simulink model "Powertrain_model"  (R2021b)
settings: Solver=VariableStepAuto  StartTime=0.0  StopTime=1220  RelTol=1e-3
values from neighbouring files (symbols this model uses):
  DR = 5.213    [Sim_script.m]    (also in workspace.mat)
  MaxLimit = [2.1951    294.39 ... (first row only)    [power_distribute_func.m]
  P_CE_idle = 0    [Sim_script.m]    (also in workspace.mat = 1)
  Trans_In = 24.086    [Sim_script.m]    (also in workspace.mat)
  w_CE_idle = 400    [Sim_script.m]    (also in workspace.mat = 32)
undefined symbols (not defined in the file or in its folder): dt, ENABLE_FUEL_CUTOFF, Fuel_con_map, H_u, P_CE_cutoff, Res_Torque, RPM_Load, T_CE_cutoff, T_CE_max, theta_CE, time, w_CE_max, w_CE_upper
libraries: visionstatistics x1, slpidlib x1
settings Model: Creator=Sagar Singhal  LastModifiedBy=Sagar Singhal

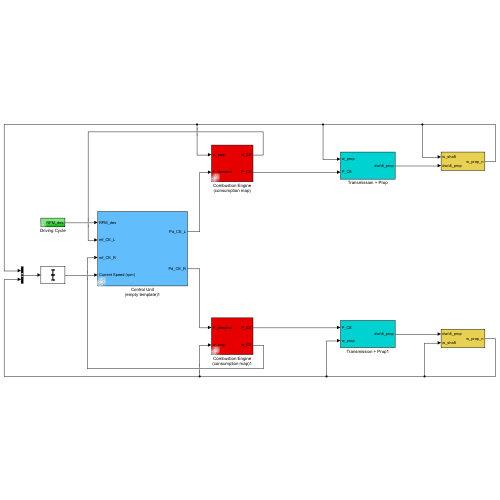
[thumbnail: Simulink's stored preview of the top-level diagram]
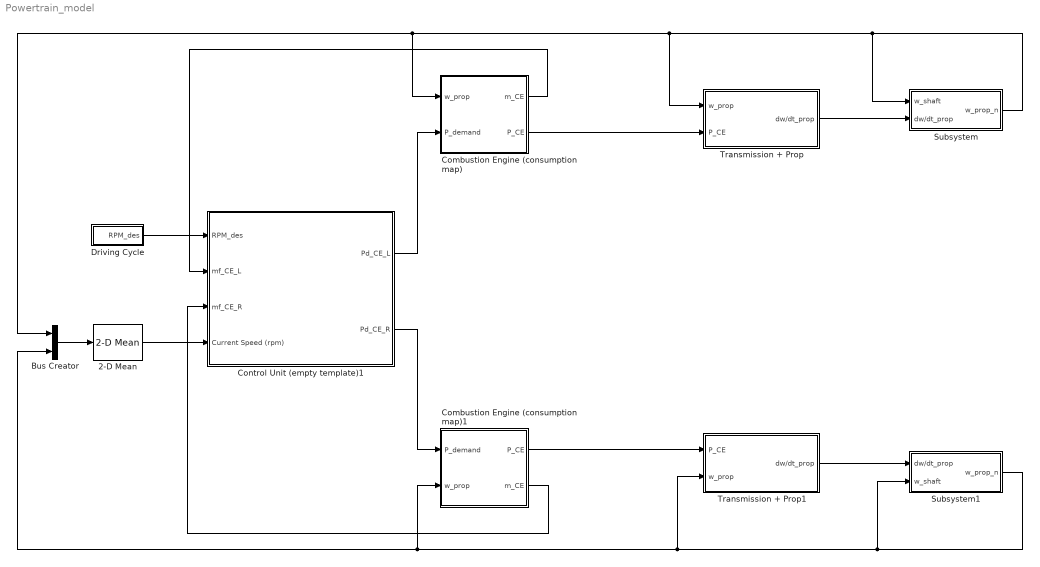
== system Powertrain_model ==
  2-D Mean : visionstatistics/2-D Mean  run=off  reset_popup=None  directionMode=Entire input  dimension=1  treatSBRowAsCol=on  outputLastDataTypeStr=Inherit: Same as accumulator  accumMode=Binary point scaling  accumWordLength=32  accumFracLength=0  accumLastDataTypeStr=fixdt([],32,0)  roiEnable=off  roiType=Rectangles  roiPortion=Entire ROI  roiOutput=Individual statistics for each ROI  roiFlag=off  roundingMode=Floor  overflowMode=off  accumDataTypeStr=fixdt([],32,0)  outputDataTypeStr=Inherit: Same as accumulator  outputMin=[]  outputMax=[]
      settings: SourceProductBaseCode=VP
  Bus Creator : BusCreator  Inputs=2
  Combustion Engine (consumption map) : Subsystem  Tag=combustion engine  AncestorBlock=|
      | qss_tb_library/Energy Converter/Combustion Engine
      | (consumption map)
  Combustion Engine (consumption map)1 : Subsystem  Tag=combustion engine  AncestorBlock=|
      | qss_tb_library/Energy Converter/Combustion Engine
      | (consumption map)
  Control Unit (empty template)1 : Subsystem  Tag=control unit  AncestorBlock=|
      | qss_tb_library/Controller/Control Unit
      | (empty template)
  Driving Cycle : Subsystem  Tag=cycle  AncestorBlock=qss_tb_library/Driving Cycle/Driving Cycle (no gradient)
  Subsystem : Subsystem
  Subsystem1 : Subsystem
  Transmission + Prop : Subsystem
  Transmission + Prop1 : Subsystem
  wires:
  Combustion Engine (consumption map)/2(P_CE) -> Transmission + Prop/2(P_CE)
  Subsystem/1(w_prop_n) -> Subsystem/1(w_shaft), Transmission + Prop/1(w_prop), Bus Creator/1, Combustion Engine (consumption map)/1(w_prop)
  Transmission + Prop/1(dw/dt_prop) -> Subsystem/2(dw/dt_prop)
  Combustion Engine (consumption map)1/1(P_CE) -> Transmission + Prop1/1(P_CE)
  Control Unit (empty template)1/2(Pd_CE_R) -> Combustion Engine (consumption map)1/1(P_demand)
  Transmission + Prop1/1(dw/dt_prop) -> Subsystem1/1(dw/dt_prop)
  Control Unit (empty template)1/1(Pd_CE_L) -> Combustion Engine (consumption map)/2(P_demand)
  Driving Cycle/1(RPM_des) -> Control Unit (empty template)1/1(RPM_des)
  Combustion Engine (consumption map)1/2(m_CE) -> Control Unit (empty template)1/3(mf_CE_R)
  Combustion Engine (consumption map)/1(m_CE) -> Control Unit (empty template)1/2(mf_CE_L)
  Bus Creator/1 -> 2-D Mean/1
  2-D Mean/1 -> Control Unit (empty template)1/4(Current Speed (rpm))
  Subsystem1/1(w_prop_n) -> Subsystem1/2(w_shaft), Transmission + Prop1/2(w_prop), Combustion Engine (consumption map)1/2(w_prop), Bus Creator/2

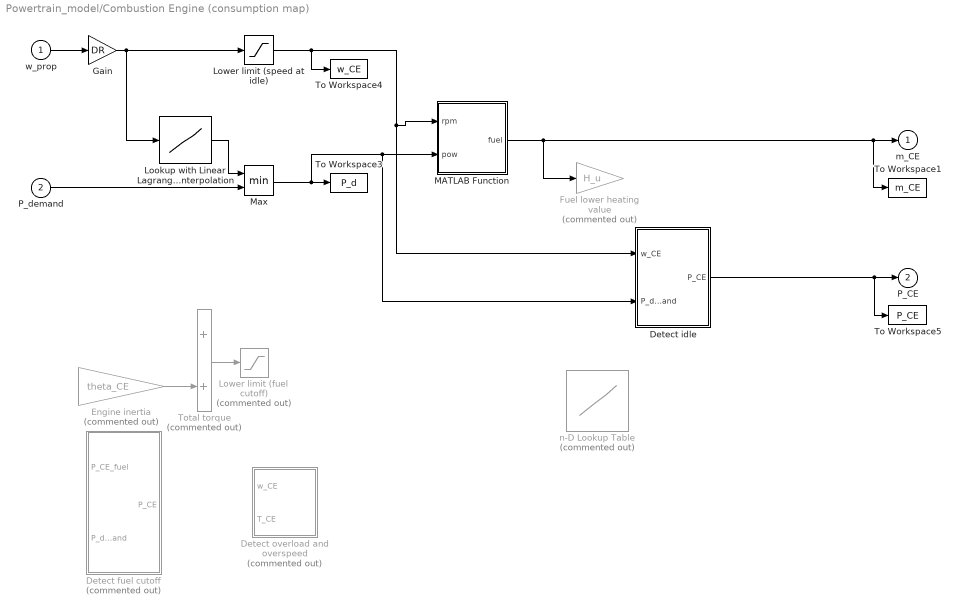
== system Powertrain_model/Combustion Engine (consumption map) ==
  w_prop : Inport
  P_demand : Inport  Port=2
  Detect fuel cutoff : Subsystem  Commented=on
  Detect idle : Subsystem
  Detect overload and overspeed : Subsystem  Commented=on
  Engine inertia : Gain  Commented=on  Gain=theta_CE  SaturateOnIntegerOverflow=on  OutDataTypeStr=Inherit: Same as input  ParamDataTypeStr=Inherit: Same as input
  Fuel lower heating value : Gain  Commented=on  Gain=H_u  SaturateOnIntegerOverflow=on  OutDataTypeStr=Inherit: Same as input  ParamDataTypeStr=Inherit: Same as input
  Gain : Gain  Gain=DR
  Lookup with Linear Lagrange Interpolation : Lookup_n-D  NumberOfTableDimensions=1  BreakpointsForDimension1=MaxLimit.('RPM')  Table=MaxLimit.('Pow_kW_')  InterpMethod=Linear Lagrange  InternalRulePriority=Speed  RndMeth=Simplest  InputSameDT=on
  Lower limit (fuel cutoff) : Saturate  Commented=on  UpperLimit=inf  LowerLimit=T_CE_cutoff
  Lower limit (speed at idle) : Saturate  UpperLimit=inf  LowerLimit=w_CE_idle
  MATLAB Function : MATLAB Function  TreatAsAtomicUnit=on
  Max : MinMax  Inputs=2
  To Workspace1 : ToWorkspace  VariableName=m_CE  SampleTime=-1
  To Workspace3 : ToWorkspace  VariableName=P_d  SampleTime=-1
  To Workspace4 : ToWorkspace  VariableName=w_CE  SampleTime=-1
  To Workspace5 : ToWorkspace  VariableName=P_CE  SampleTime=-1
  Total torque : Sum  Commented=on  InputSameDT=on  SaturateOnIntegerOverflow=on  OutDataTypeStr=Inherit: Same as first input
  n-D Lookup Table : Lookup_n-D  Commented=on  LookupTableObject=''  BreakpointsForDimension1=Fuel_con_map.('RPM')  BreakpointsForDimension2=Fuel_con_map.('Power(kW)')  BreakpointsForDimension3=[5, 7]  BreakpointsForDimension1FirstPoint=10  BreakpointsForDimension2FirstPoint=10  BreakpointsForDimension1Spacing=12  BreakpointsForDimension2Spacing=12  IndexSearchMethod=Evenly spaced points  Table=Fuel_con_map.('Fuel(g/KWh)')  InterpMethod=Cubic spline  ExtrapMethod=Cubic spline  DiagnosticForOutOfRangeInput=Error  InternalRulePriority=Speed  RndMeth=Simplest  InputSameDT=on
      settings: InputPortMap=u0,u1
  m_CE : Outport  InitialOutput=0
  P_CE : Outport  Port=2  InitialOutput=0
  wires:
  Max/1 -> MATLAB Function/2(pow), Detect idle/2(P_demand), To Workspace3/1
  MATLAB Function/1(fuel) -> To Workspace1/1, m_CE/1, Fuel lower heating value/1
  w_prop/1 -> Gain/1
  Lower limit (speed at idle)/1 -> To Workspace4/1, MATLAB Function/1(rpm), Detect idle/1(w_CE)
  Engine inertia/1 -> Total torque/2
  Total torque/1 -> Lower limit (fuel cutoff)/1
  ? -> Engine inertia/1
  ? -> Total torque/1
  Detect idle/1(P_CE) -> To Workspace5/1, P_CE/1
  P_demand/1 -> Max/2
  Lookup with Linear Lagrange Interpolation/1 -> Max/1
  Gain/1 -> Lookup with Linear Lagrange Interpolation/1, Lower limit (speed at idle)/1

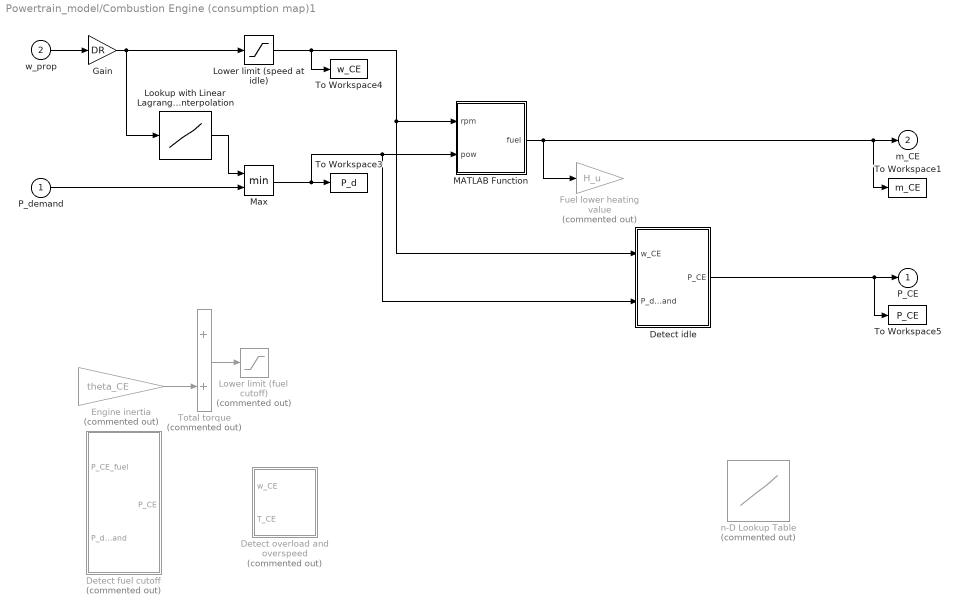
== system Powertrain_model/Combustion Engine (consumption map)1 ==
  P_demand : Inport
  w_prop : Inport  Port=2
  Detect fuel cutoff : Subsystem  Commented=on
  Detect idle : Subsystem
  Detect overload and overspeed : Subsystem  Commented=on
  Engine inertia : Gain  Commented=on  Gain=theta_CE  SaturateOnIntegerOverflow=on  OutDataTypeStr=Inherit: Same as input  ParamDataTypeStr=Inherit: Same as input
  Fuel lower heating value : Gain  Commented=on  Gain=H_u  SaturateOnIntegerOverflow=on  OutDataTypeStr=Inherit: Same as input  ParamDataTypeStr=Inherit: Same as input
  Gain : Gain  Gain=DR
  Lookup with Linear Lagrange Interpolation : Lookup_n-D  NumberOfTableDimensions=1  BreakpointsForDimension1=MaxLimit.('RPM')  Table=MaxLimit.('Pow_kW_')  InterpMethod=Linear Lagrange  InternalRulePriority=Speed  RndMeth=Simplest  InputSameDT=on
  Lower limit (fuel cutoff) : Saturate  Commented=on  UpperLimit=inf  LowerLimit=T_CE_cutoff
  Lower limit (speed at idle) : Saturate  UpperLimit=inf  LowerLimit=w_CE_idle
  MATLAB Function : MATLAB Function  TreatAsAtomicUnit=on
  Max : MinMax  Inputs=2
  To Workspace1 : ToWorkspace  VariableName=m_CE  SampleTime=-1
  To Workspace3 : ToWorkspace  VariableName=P_d  SampleTime=-1
  To Workspace4 : ToWorkspace  VariableName=w_CE  SampleTime=-1
  To Workspace5 : ToWorkspace  VariableName=P_CE  SampleTime=-1
  Total torque : Sum  Commented=on  InputSameDT=on  SaturateOnIntegerOverflow=on  OutDataTypeStr=Inherit: Same as first input
  n-D Lookup Table : Lookup_n-D  Commented=on  LookupTableObject=''  BreakpointsForDimension1=Fuel_con_map.('RPM')  BreakpointsForDimension2=Fuel_con_map.('Power(kW)')  BreakpointsForDimension3=[5, 7]  BreakpointsForDimension1FirstPoint=10  BreakpointsForDimension2FirstPoint=10  BreakpointsForDimension1Spacing=12  BreakpointsForDimension2Spacing=12  IndexSearchMethod=Evenly spaced points  Table=Fuel_con_map.('Fuel(g/KWh)')  InterpMethod=Cubic spline  ExtrapMethod=Cubic spline  DiagnosticForOutOfRangeInput=Error  InternalRulePriority=Speed  RndMeth=Simplest  InputSameDT=on
      settings: InputPortMap=u0,u1
  P_CE : Outport  InitialOutput=0
  m_CE : Outport  Port=2  InitialOutput=0
  wires:
  Max/1 -> MATLAB Function/2(pow), Detect idle/2(P_demand), To Workspace3/1
  MATLAB Function/1(fuel) -> To Workspace1/1, m_CE/1, Fuel lower heating value/1
  w_prop/1 -> Gain/1
  Lower limit (speed at idle)/1 -> To Workspace4/1, MATLAB Function/1(rpm), Detect idle/1(w_CE)
  Engine inertia/1 -> Total torque/2
  Total torque/1 -> Lower limit (fuel cutoff)/1
  ? -> Engine inertia/1
  ? -> Total torque/1
  Detect idle/1(P_CE) -> To Workspace5/1, P_CE/1
  P_demand/1 -> Max/2
  Lookup with Linear Lagrange Interpolation/1 -> Max/1
  Gain/1 -> Lookup with Linear Lagrange Interpolation/1, Lower limit (speed at idle)/1

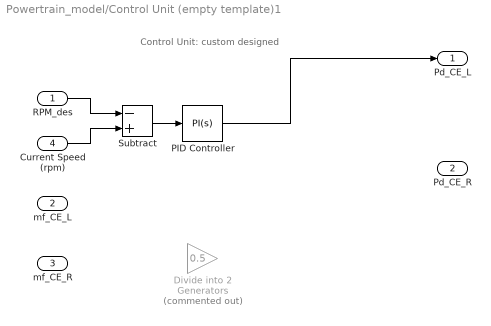
== system Powertrain_model/Control Unit (empty template)1 ==
  note: Control Unit: custom designed
  RPM_des : Inport
  mf_CE_L : Inport  Port=2
  mf_CE_R : Inport  Port=3
  Current Speed (rpm) : Inport  Port=4
  Divide into 2 Generators : Gain  Commented=on  Gain=0.5
  PID Controller : slpidlib/PID Controller  Controller=PI  Form=Parallel  TimeDomain=Continuous-time  UseExternalTs=off  SampleTime=-1  IntegratorMethod=Forward Euler  FilterMethod=Forward Euler  ControllerParametersSource=internal  P=4  I=1.2  D=0  UseFilter=on  N=100  TunerSelectOption=Transfer Function Based (PID Tuner App)  InitialConditionSource=internal  InitialConditionForIntegrator=0  InitialConditionForFilter=0  DifferentiatorICPrevScaledInput=0  ExternalReset=none  TrackingMode=off  Kt=1  LimitOutput=off  SatLimitsSource=internal  UpperSaturationLimit=inf  LowerSaturationLimit=-inf  LinearizeAsGain=on  AntiWindupMode=none  Kb=1  POutMin=[]  POutMax=[]  IOutMin=[]  IOutMax=[]  DOutMin=[]  DOutMax=[]  NOutMin=[]  NOutMax=[]  SumOutMin=[]  SumOutMax=[]  SaturationOutMin=[]  SaturationOutMax=[]  PParamMin=[]  PParamMax=[]  IParamMin=[]  IParamMax=[]  DParamMin=[]  DParamMax=[]  NParamMin=[]  NParamMax=[]  KbParamMin=[]  KbParamMax=[]  KtParamMin=[]  KtParamMax=[]  KbOutMin=[]  KbOutMax=[]  KtOutMin=[]  KtOutMax=[]  IntegratorOutMin=[]  IntegratorOutMax=[]  FilterOutMin=[]  FilterOutMax=[]  SumI1OutMin=[]  SumI1OutMax=[]  SumI2OutMin=[]  SumI2OutMax=[]  SumI3OutMin=[]  SumI3OutMax=[]  SumI4OutMin=[]  SumI4OutMax=[]  SumDOutMin=[]  SumDOutMax=[]  DifferentiatorOutMin=[]  DifferentiatorOutMax=[]  FilterDiffOutCoefMin=[]  FilterDiffOutCoefMax=[]  ReciprocalOutMin=[]  ReciprocalOutMax=[]  SumDenOutMin=[]  SumDenOutMax=[]  SumNumOutMin=[]  SumNumOutMax=[]  DivideOutMin=[]  DivideOutMax=[]  UdiffTsProdOutMin=[]  UdiffTsProdOutMax=[]  NTsProdOutMin=[]  NTsProdOutMax=[]  UintegralTsProdOutMin=[]  UintegralTsProdOutMax=[]  UngainTsProdOutMin=[]  UngainTsProdOutMax=[]  IntegratorContinuousStateAttributes=''  IntegratorStateMustResolveToSignalObject=off  IntegratorRTWStateStorageClass=Auto  FilterContinuousStateAttributes=''  FilterStateMustResolveToSignalObject=off  FilterRTWStateStorageClass=Auto  ParallelPVariant=InternalParameters  IdealPVariant=Disabled  IVariant=InternalParameters  DVariant=Disabled  IntegratorVariant=Continuous  SatVariant=Disabled  AWVariant=Passthrough  PCopyVariant=Disabled  TRVariant=Disabled  FdbkBlocksVariant=Forward  IdealPFdbkVariant=Disabled  SatFdbkVariant=Disabled  DerivativeFilterVariant=Disabled  NVariant=Disabled  NCopyVariant=Disabled_SignalSpec  FilterICVariant=Disabled  IntegratorICVariant=InternalICs  ExternalResetVariant=Disabled  TRSumVariant=Passthrough  SumFdbkVariant=Disabled  SumVariant=Sum_PI  TsampFilterVariant=InternalTs  TsampNgainVariant=Passthrough  TsampIntegralVariant=Passthrough  ExternalSaturationOutDataTypeStr=Inherit: Same as second input
  Subtract : Sum  Inputs=-+
  Pd_CE_L : Outport  InitialOutput=0
  Pd_CE_R : Outport  Port=2  InitialOutput=0
  wires:
  Current Speed (rpm)/1 -> Subtract/2
  RPM_des/1 -> Subtract/1
  PID Controller/1 -> Pd_CE_L/1
  Subtract/1 -> PID Controller/1

== system Powertrain_model/Driving Cycle ==
  1-D Lookup Table : Lookup_n-D  NumberOfTableDimensions=1  BreakpointsForDimension1=time  Table=RPM_Load  InternalRulePriority=Speed  RndMeth=Simplest  InputSameDT=on
  Clock : Clock
  To Workspace1 : ToWorkspace  VariableName=t  SampleTime=-1
  RPM_des : Outport
  wires:
  Clock/1 -> 1-D Lookup Table/1, To Workspace1/1
  1-D Lookup Table/1 -> RPM_des/1

== system Powertrain_model/Subsystem ==
  w_shaft : Inport
  dw/dt_prop : Inport  Port=2
  Add : Sum
  Gain : Gain  Gain=1/DR
  time_step : Gain  Gain=dt
  w_prop_n : Outport
  wires:
  dw/dt_prop/1 -> time_step/1
  time_step/1 -> Add/2
  w_shaft/1 -> Gain/1
  Add/1 -> w_prop_n/1
  Gain/1 -> Add/1

== system Powertrain_model/Subsystem1 ==
  dw/dt_prop : Inport
  w_shaft : Inport  Port=2
  Add : Sum
  Gain : Gain  Gain=1/DR
  time_step : Gain  Gain=dt
  w_prop_n : Outport
  wires:
  dw/dt_prop/1 -> time_step/1
  time_step/1 -> Add/2
  w_shaft/1 -> Gain/1
  Add/1 -> w_prop_n/1
  Gain/1 -> Add/1

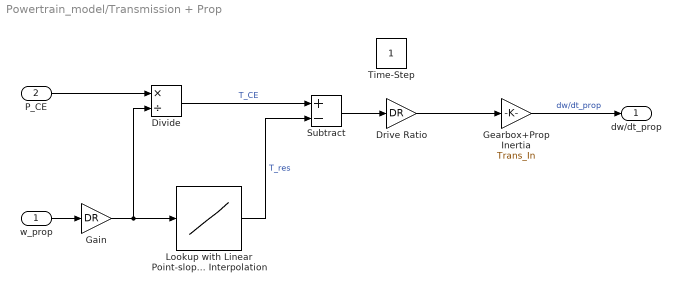
== system Powertrain_model/Transmission + Prop ==
  w_prop : Inport
  P_CE : Inport  Port=2
  Divide : Product  Inputs=*/
  Drive Ratio : Gain  Gain=DR
  Gain : Gain  Gain=DR
  Gearbox+Prop Inertia : Gain  Gain=Trans_In
  Lookup with Linear Point-slope Interpolation : Lookup_n-D  NumberOfTableDimensions=1  BreakpointsForDimension1=Res_Torque.('RPMEngine')  Table=Res_Torque.('TorqueNM')  InternalRulePriority=Speed  RndMeth=Simplest  InputSameDT=on
  Subtract : Sum  Inputs=+-
  Time-Step : Constant
  dw/dt_prop : Outport
  wires:
  Lookup with Linear Point-slope Interpolation/1 -> Subtract/2  "T_res"
  P_CE/1 -> Divide/1
  Subtract/1 -> Drive Ratio/1
  Gearbox+Prop Inertia/1 -> dw/dt_prop/1  "dw/dt_prop"
  w_prop/1 -> Gain/1
  Drive Ratio/1 -> Gearbox+Prop Inertia/1
  Divide/1 -> Subtract/1  "T_CE"
  Gain/1 -> Divide/2, Lookup with Linear Point-slope Interpolation/1

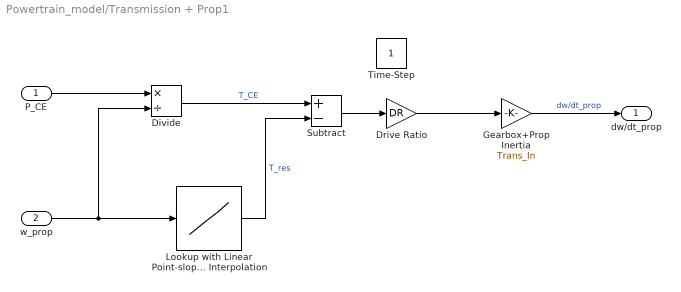
== system Powertrain_model/Transmission + Prop1 ==
  P_CE : Inport
  w_prop : Inport  Port=2
  Divide : Product  Inputs=*/
  Drive Ratio : Gain  Gain=DR
  Gearbox+Prop Inertia : Gain  Gain=Trans_In
  Lookup with Linear Point-slope Interpolation : Lookup_n-D  NumberOfTableDimensions=1  BreakpointsForDimension1=Res_Torque.('RPMEngine')  Table=Res_Torque.('TorqueNM')  InternalRulePriority=Speed  RndMeth=Simplest  InputSameDT=on
  Subtract : Sum  Inputs=+-
  Time-Step : Constant
  dw/dt_prop : Outport
  wires:
  Lookup with Linear Point-slope Interpolation/1 -> Subtract/2  "T_res"
  P_CE/1 -> Divide/1
  Subtract/1 -> Drive Ratio/1
  Gearbox+Prop Inertia/1 -> dw/dt_prop/1  "dw/dt_prop"
  w_prop/1 -> Divide/2, Lookup with Linear Point-slope Interpolation/1
  Drive Ratio/1 -> Gearbox+Prop Inertia/1
  Divide/1 -> Subtract/1  "T_CE"

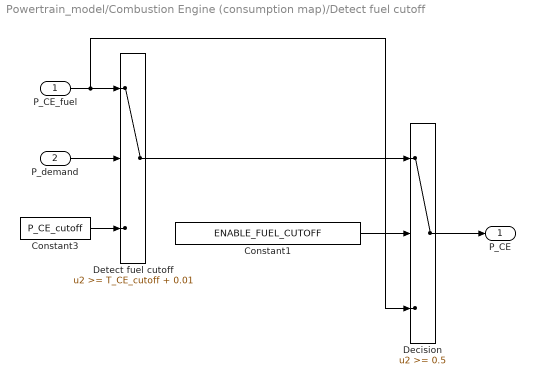
== system Powertrain_model/Combustion Engine (consumption map)/Detect fuel cutoff ==
  P_CE_fuel : Inport
  P_demand : Inport  Port=2
  Constant1 : Constant  Value=ENABLE_FUEL_CUTOFF
  Constant3 : Constant  Value=P_CE_cutoff
  Decision : Switch  Threshold=0.5
  Detect fuel cutoff : Switch  Threshold=T_CE_cutoff + 0.01  SaturateOnIntegerOverflow=on  InputSameDT=on
  P_CE : Outport
  wires:
  Decision/1 -> P_CE/1
  Constant1/1 -> Decision/2
  Detect fuel cutoff/1 -> Decision/1
  P_CE_fuel/1 -> Decision/3, Detect fuel cutoff/1
  P_demand/1 -> Detect fuel cutoff/2
  Constant3/1 -> Detect fuel cutoff/3

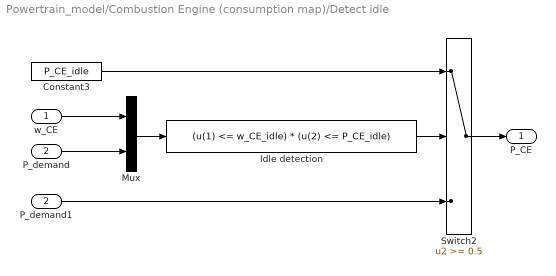
== system Powertrain_model/Combustion Engine (consumption map)/Detect idle ==
  w_CE : Inport
  P_demand : Inport  Port=2
  Constant3 : Constant  Value=P_CE_idle
  Idle detection : Fcn  Expr=(u(1) <= w_CE_idle) * (u(2) <= P_CE_idle)
  Mux : Mux  Inputs=2
  P_demand1 : InportShadow  Port=2
  Switch2 : Switch  Threshold=0.5  SaturateOnIntegerOverflow=on  InputSameDT=on
  P_CE : Outport  InitialOutput=0
  wires:
  Constant3/1 -> Switch2/1
  Switch2/1 -> P_CE/1
  P_demand1/1 -> Switch2/3
  Idle detection/1 -> Switch2/2
  w_CE/1 -> Mux/1
  P_demand/1 -> Mux/2
  Mux/1 -> Idle detection/1

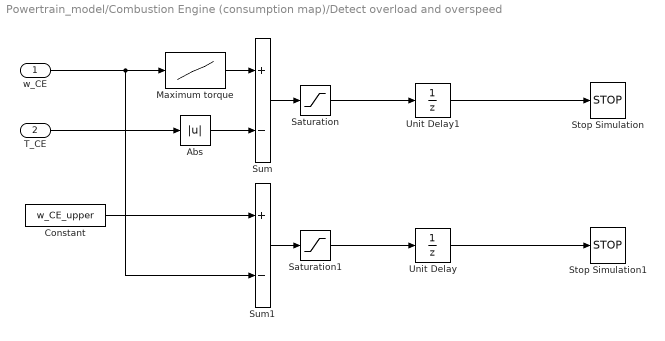
== system Powertrain_model/Combustion Engine (consumption map)/Detect overload and overspeed ==
  w_CE : Inport
  T_CE : Inport  Port=2
  Abs : Abs  SaturateOnIntegerOverflow=on
  Constant : Constant  Value=w_CE_upper
  Maximum torque : Lookup  InputValues=w_CE_max  Table=T_CE_max  SaturateOnIntegerOverflow=on
  Saturation : Saturate  UpperLimit=0  LowerLimit=-inf
  Saturation1 : Saturate  UpperLimit=0  LowerLimit=-inf
  Stop Simulation : Stop
  Stop Simulation1 : Stop
  Sum : Sum  Inputs=+-  InputSameDT=on  SaturateOnIntegerOverflow=on  OutDataTypeStr=Inherit: Same as first input
  Sum1 : Sum  Inputs=+-  InputSameDT=on  SaturateOnIntegerOverflow=on  OutDataTypeStr=Inherit: Same as first input
  Unit Delay : UnitDelay  SampleTime=-1  HasFrameUpgradeWarning=on
  Unit Delay1 : UnitDelay  SampleTime=-1  HasFrameUpgradeWarning=on
  wires:
  Unit Delay1/1 -> Stop Simulation/1
  Unit Delay/1 -> Stop Simulation1/1
  Saturation1/1 -> Unit Delay/1
  Sum1/1 -> Saturation1/1
  Constant/1 -> Sum1/1
  Saturation/1 -> Unit Delay1/1
  Abs/1 -> Sum/2
  Maximum torque/1 -> Sum/1
  T_CE/1 -> Abs/1
  w_CE/1 -> Sum1/2, Maximum torque/1
  Sum/1 -> Saturation/1

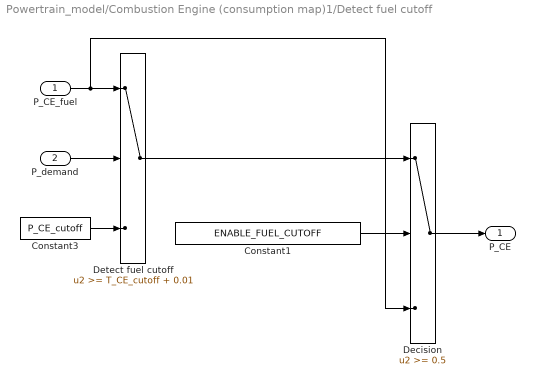
== system Powertrain_model/Combustion Engine (consumption map)1/Detect fuel cutoff ==
  P_CE_fuel : Inport
  P_demand : Inport  Port=2
  Constant1 : Constant  Value=ENABLE_FUEL_CUTOFF
  Constant3 : Constant  Value=P_CE_cutoff
  Decision : Switch  Threshold=0.5
  Detect fuel cutoff : Switch  Threshold=T_CE_cutoff + 0.01  SaturateOnIntegerOverflow=on  InputSameDT=on
  P_CE : Outport
  wires:
  Decision/1 -> P_CE/1
  Constant1/1 -> Decision/2
  Detect fuel cutoff/1 -> Decision/1
  P_CE_fuel/1 -> Decision/3, Detect fuel cutoff/1
  P_demand/1 -> Detect fuel cutoff/2
  Constant3/1 -> Detect fuel cutoff/3

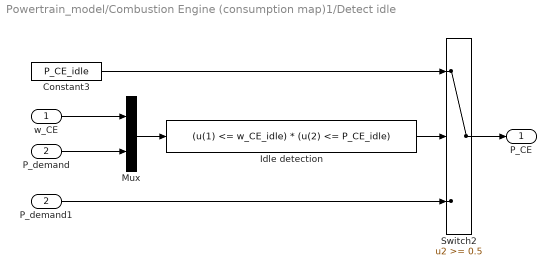
== system Powertrain_model/Combustion Engine (consumption map)1/Detect idle ==
  w_CE : Inport
  P_demand : Inport  Port=2
  Constant3 : Constant  Value=P_CE_idle
  Idle detection : Fcn  Expr=(u(1) <= w_CE_idle) * (u(2) <= P_CE_idle)
  Mux : Mux  Inputs=2
  P_demand1 : InportShadow  Port=2
  Switch2 : Switch  Threshold=0.5  SaturateOnIntegerOverflow=on  InputSameDT=on
  P_CE : Outport  InitialOutput=0
  wires:
  Constant3/1 -> Switch2/1
  Switch2/1 -> P_CE/1
  P_demand1/1 -> Switch2/3
  Idle detection/1 -> Switch2/2
  w_CE/1 -> Mux/1
  P_demand/1 -> Mux/2
  Mux/1 -> Idle detection/1

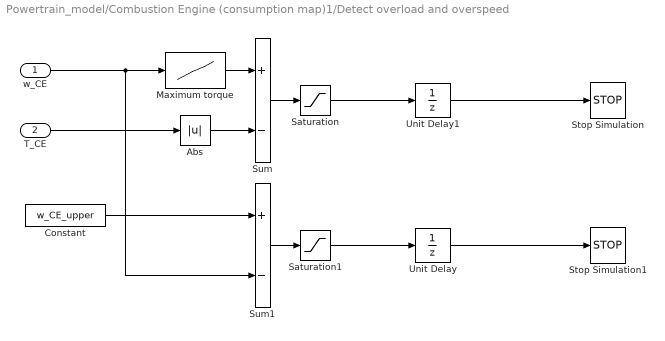
== system Powertrain_model/Combustion Engine (consumption map)1/Detect overload and overspeed ==
  w_CE : Inport
  T_CE : Inport  Port=2
  Abs : Abs  SaturateOnIntegerOverflow=on
  Constant : Constant  Value=w_CE_upper
  Maximum torque : Lookup  InputValues=w_CE_max  Table=T_CE_max  SaturateOnIntegerOverflow=on
  Saturation : Saturate  UpperLimit=0  LowerLimit=-inf
  Saturation1 : Saturate  UpperLimit=0  LowerLimit=-inf
  Stop Simulation : Stop
  Stop Simulation1 : Stop
  Sum : Sum  Inputs=+-  InputSameDT=on  SaturateOnIntegerOverflow=on  OutDataTypeStr=Inherit: Same as first input
  Sum1 : Sum  Inputs=+-  InputSameDT=on  SaturateOnIntegerOverflow=on  OutDataTypeStr=Inherit: Same as first input
  Unit Delay : UnitDelay  SampleTime=-1  HasFrameUpgradeWarning=on
  Unit Delay1 : UnitDelay  SampleTime=-1  HasFrameUpgradeWarning=on
  wires:
  Unit Delay1/1 -> Stop Simulation/1
  Unit Delay/1 -> Stop Simulation1/1
  Saturation1/1 -> Unit Delay/1
  Sum1/1 -> Saturation1/1
  Constant/1 -> Sum1/1
  Saturation/1 -> Unit Delay1/1
  Abs/1 -> Sum/2
  Maximum torque/1 -> Sum/1
  T_CE/1 -> Abs/1
  w_CE/1 -> Sum1/2, Maximum torque/1
  Sum/1 -> Saturation/1

== matlab function Powertrain_model/Combustion Engine (consumption map)/MATLAB Function ==
  data: rpm input; fuel output; pow input
function fuel  = fuel_con_map(rpm,pow)
x = rpm;
y = pow;
p00 =         203;
p10 =      0.9394;
p01 =      -8.327;
p20 =       1.894;
p11 =     -0.7168;
p02 =       1.321;
p30 =      0.2621;
p21 =       1.482;
p12 =       5.529;
p03 =      -2.619;
p40 =      0.9252;
p31 =      -3.236;
p22 =       3.413;
p13 =      -2.546;
p04 =        2.97;
p50 =     -0.1717;
p41 =       1.492;
p32 =      -2.908;
p23 =      0.2029;
p14 =      0.4508;
p05 =     -0.7973;
fuel = p00 + p10*x + p01*y + p20*x^2 + p11*x*y + p02*y^2 + p30*x^3 + p21*x^2*y ...
         + p12*x*y^2 + p03*y^3 + p40*x^4 + p31*x^3*y + p22*x^2*y^2 ...
         + p13*x*y^3 + p04*y^4 + p50*x^5 + p41*x^4*y + p32*x^3*y^2 ...
          + p23*x^2*y^3 + p14*x*y^4 + p05*y^5;
end

== matlab function Powertrain_model/Combustion Engine (consumption map)1/MATLAB Function ==
  data: rpm input; fuel output; pow input
function fuel  = fuel_con_map(rpm,pow)
x = rpm;
y = pow;
p00 =         203;
p10 =      0.9394;
p01 =      -8.327;
p20 =       1.894;
p11 =     -0.7168;
p02 =       1.321;
p30 =      0.2621;
p21 =       1.482;
p12 =       5.529;
p03 =      -2.619;
p40 =      0.9252;
p31 =      -3.236;
p22 =       3.413;
p13 =      -2.546;
p04 =        2.97;
p50 =     -0.1717;
p41 =       1.492;
p32 =      -2.908;
p23 =      0.2029;
p14 =      0.4508;
p05 =     -0.7973;
fuel = p00 + p10*x + p01*y + p20*x^2 + p11*x*y + p02*y^2 + p30*x^3 + p21*x^2*y ...
         + p12*x*y^2 + p03*y^3 + p40*x^4 + p31*x^3*y + p22*x^2*y^2 ...
         + p13*x*y^3 + p04*y^4 + p50*x^5 + p41*x^4*y + p32*x^3*y^2 ...
          + p23*x^2*y^3 + p14*x*y^4 + p05*y^5;
end
